simulink library "torque_2_rpm_lib"  (R2018b)
settings: Solver=VariableStepAuto  StartTime=0.0  StopTime=10.0  RelTol=1e-3
undefined symbols (not defined in the file or in its folder): DiscIntNeverNeededParam, fswParams
settings Model: Creator=Taylor  LastModifiedBy=taylorreynolds

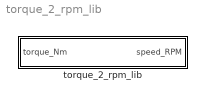
== system torque_2_rpm_lib ==
  torque_2_rpm_lib : Subsystem  TreatAsAtomicUnit=on
      settings: RTWFcnNameOpts=Use subsystem name  RTWFileNameOpts=Use subsystem name

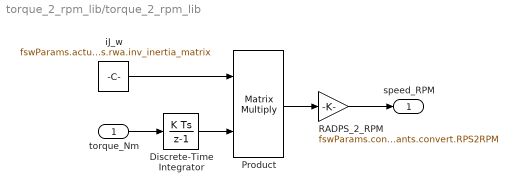
== system torque_2_rpm_lib/torque_2_rpm_lib ==
  torque_Nm : Inport
  Discrete-Time Integrator : DiscreteIntegrator  InitialCondition=fswParams.actuators.rwa.ic.momentum  SampleTime=-1  ICPrevOutput=DiscIntNeverNeededParam  ICPrevScaledInput=DiscIntNeverNeededParam
  Product : Product  Multiplication=Matrix(*)
  RADPS_2_RPM : Gain  Gain=fswParams.constants.convert.RPS2RPM
  iJ_w : Constant  Value=fswParams.actuators.rwa.inv_inertia_matrix
  speed_RPM : Outport
  wires:
  torque_Nm/1 -> Discrete-Time Integrator/1
  iJ_w/1 -> Product/1
  Product/1 -> RADPS_2_RPM/1
  RADPS_2_RPM/1 -> speed_RPM/1
  Discrete-Time Integrator/1 -> Product/2
